simulink model "gm_PN_generator_Tx_interface"  (R2020a)
settings: Solver=FixedStepDiscrete  StartTime=0.0  StopTime=10  RelTol=1e-3  EnableMultiTasking=on
undefined symbols (not defined in the file): AXI4, Fs, ip, Lite, usb
libraries: axiinterfacelib x6, commfilt2 x4, plutoradiolib x2, commdigbbndpm3 x2, commseqgen3 x1, commutil2 x1
settings Model: Creator=juanj  LastModifiedBy=juanj
settings SolverCC: PositivePriorityOrder=on
settings OptimizationCC: BlockReduction=off  ConditionallyExecuteInputs=off  EnhancedBackFolding=on  PassReuseOutputArgsAs=Individual arguments  ZeroExternalMemoryAtStartup=off  ZeroInternalMemoryAtStartup=off  MaxStackSize=64  OptimizeBlockOrder=speed  DifferentSizesBufferReuse=on  OptimizationCustomize=off  EfficientTunableParamExpr=on
settings DebuggingCC: SignalRangeChecking=warning  AlgebraicLoopMsg=error  SingleTaskRateTransMsg=error  ParameterTunabilityLossMsg=error  UnderSpecifiedDimensionMsg=warning
settings HardwareCC: ProdBitPerPointer=32  ProdBitPerSizeT=32  ProdBitPerPtrDiffT=32  ProdLargestAtomicInteger=Long  ProdLargestAtomicFloat=Double  ProdWordSize=32  ProdLongLongMode=on  ProdHWDeviceType=ARM Compatible->ARM Cortex  TargetBitPerPointer=64  TargetBitPerSizeT=64  TargetBitPerPtrDiffT=64  TargetLongLongMode=on  TargetIntDivRoundTo=Zero  TargetEndianess=LittleEndian  TargetWordSize=64  TargetHWDeviceType=Custom Processor->MATLAB Host Computer
settings SFSimCC: MATLABDynamicMemAlloc=off
settings RTWCC: SystemTargetFile=ert.tlc  HardwareBoard=ZedBoard  TemplateMakefile=ert_default_tmf  Toolchain=Linaro AArch32 Linux v6.3.1
settings CodeAppCC: ForceParamTrailComments=on  IgnoreCustomStorageClasses=off  OperatorAnnotations=on  SimulinkDataObjDesc=on  SFDataObjDesc=on  InsertBlockDesc=on

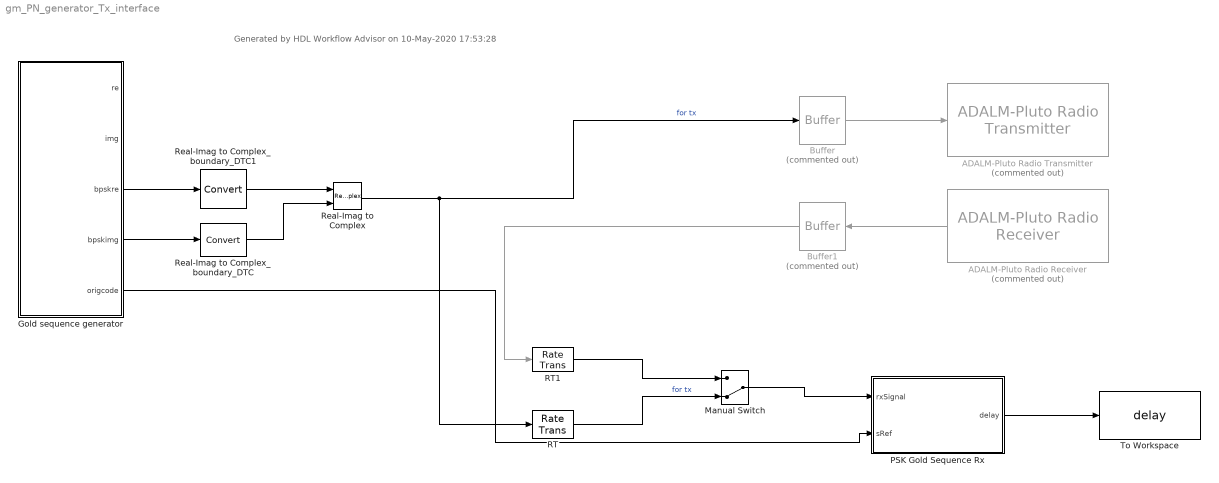
== system gm_PN_generator_Tx_interface ==
  note: Generated by HDL Workflow Advisor on 10-May-2020 17:53:28
  ADALM-Pluto Radio Receiver : plutoradiolib/ADALM-Pluto Radio Receiver  Commented=on  RadioID=usb:0  uri=ip:10.0.0.200  CenterFrequencySource=Dialog  CenterFrequency=900e6  GainSource=AGC Slow Attack  GainSourceBlock=AGC Slow Attack  Gain=10  ChannelMapping=1  BasebandSampleRate=0.5e6  OutputDataType=double  SamplesPerFrame=11216  OverflowOutputPort=off  EnableBurstMode=off  NumFramesInBurst=1  ShowAdvancedProperties=off  UseCustomFilter=off  filtPathRates=[737280000 11520000 3840000 1920000 960000 240000]  filtCoefficients=[-192 82 85 -215 228 -102 -110 290 -318 145 160 -426 471 -215 -238 633 -697 318 349 -923 1009 -457 -498 1309 -1423 640 693 -1812 1959 -876 -945 2458 -2647 1180 1268 -3290 3534 -1572 -1688 4375 -4698 2091 2247 -5836 6284 -2807 -3031 7918 -8588 3870 4225 -11182 12324 -5662 -6330 17255 -19735 9507 11312 -33568 43355 -25227 -42139 305542 305542 -42139 -25227 43355 -33568 11312 9507 -19735 17255 -6330 -5662 12324 -11182 4225 3870 -8588 7918 -3031 -2807 6284 -5836 2247 2091 -4698 4375 -1688 -1572 3534 -3290 1268 1180 -2647 2458 -945 -876 1959 -1812 693 640 -1423 1309 -498 -457 1009 -923 349 318 -697 633 -238 -215 471 -426 160 145 -318 290 -110 -102 228 -215 85 82 -192]  filtCoefficientSize=128  filtDecimInterpFactor=4  filtGain=-12  filtRFBandwidth=18000000  filterConfigStruct=struct()  EnableQuadratureCorrection=on  EnableRFDCCorrection=on  EnableBasebandDCCorrection=on  FrequencyCorrection=0  OverrideSampleTime=off  SampleTime=0.02  DataTimeout=Inf  ENSMPinControlMode=None  BISTLoopbackMode=Disabled  BISTToneInject=Disabled  BISTSignalGen=PRBS  BISTToneFreq=Fs/32  BISTToneLevel=0
      settings: SourceProductBaseCode=PLUTO
  ADALM-Pluto Radio Transmitter : plutoradiolib/ADALM-Pluto Radio Transmitter  Commented=on  RadioID=usb:0  uri=ip:10.0.0.200  CenterFrequencySource=Dialog  CenterFrequency=900e6  GainSource=Dialog  Gain=0  ChannelMapping=1  BasebandSampleRate=0.5e6  UnderflowOutputPort=off  ShowAdvancedProperties=off  UseCustomFilter=off  filtPathRates=[737280000 11520000 3840000 1920000 960000 240000]  filtCoefficients=[-192 82 85 -215 228 -102 -110 290 -318 145 160 -426 471 -215 -238 633 -697 318 349 -923 1009 -457 -498 1309 -1423 640 693 -1812 1959 -876 -945 2458 -2647 1180 1268 -3290 3534 -1572 -1688 4375 -4698 2091 2247 -5836 6284 -2807 -3031 7918 -8588 3870 4225 -11182 12324 -5662 -6330 17255 -19735 9507 11312 -33568 43355 -25227 -42139 305542 305542 -42139 -25227 43355 -33568 11312 9507 -19735 17255 -6330 -5662 12324 -11182 4225 3870 -8588 7918 -3031 -2807 6284 -5836 2247 2091 -4698 4375 -1688 -1572 3534 -3290 1268 1180 -2647 2458 -945 -876 1959 -1812 693 640 -1423 1309 -498 -457 1009 -923 349 318 -697 633 -238 -215 471 -426 160 145 -318 290 -110 -102 228 -215 85 82 -192]  filtCoefficientSize=128  filtDecimInterpFactor=4  filtGain=-12  filtRFBandwidth=18000000  filterConfigStruct=struct()  DataSourceSelect=Input Port  DDSTone1Freq=5e3  DDSTone2Freq=10e3  DDSTone1Scale=0.5  DDSTone2Scale=0.25  DataTimeout=Inf  FrequencyCorrection=0  ENSMPinControlMode=None  BISTLoopbackMode=Disabled  BISTToneInject=Disabled  BISTSignalGen=PRBS  BISTToneFreq=Fs/32  BISTToneLevel=0
      settings: SourceProductBaseCode=PLUTO
  Buffer : Buffer  Commented=on  N=11216  OutputFrames=off
  Buffer1 : Buffer  Commented=on  N=1  OutputFrames=off
  Gold sequence generator : Subsystem  TreatAsAtomicUnit=on
  Manual Switch : ManualSwitch  CurrentSetting=0
  PSK Gold Sequence Rx : Subsystem
  RT : RateTransition  OutPortSampleTime=5e-07
  RT1 : RateTransition  OutPortSampleTime=5e-07
  Real-Imag to Complex : RealImagToComplex
  Real-Imag to Complex_boundary_DTC : DataTypeConversion  SaturateOnIntegerOverflow=on  RndMeth=Zero
  Real-Imag to Complex_boundary_DTC1 : DataTypeConversion  SaturateOnIntegerOverflow=on  RndMeth=Zero
  To Workspace : ToWorkspace  VariableName=delay  SampleTime=-1
      settings: Save2DSignal=2-D array (concatenate along first dimension)
  wires:
  RT1/1 -> Manual Switch/1
  Buffer1/1 -> RT1/1
  ADALM-Pluto Radio Receiver/1 -> Buffer1/1
  RT/1 -> Manual Switch/2  "for tx"
  Manual Switch/1 -> PSK Gold Sequence Rx/1(rxSignal)
  PSK Gold Sequence Rx/1(delay) -> To Workspace/1
  Gold sequence generator/5(origcode) -> PSK Gold Sequence Rx/2(sRef)
  Real-Imag to Complex_boundary_DTC1/1 -> Real-Imag to Complex/1
  Gold sequence generator/3(bpskre) -> Real-Imag to Complex_boundary_DTC1/1
  Real-Imag to Complex_boundary_DTC/1 -> Real-Imag to Complex/2
  Gold sequence generator/4(bpskimg) -> Real-Imag to Complex_boundary_DTC/1
  Buffer/1 -> ADALM-Pluto Radio Transmitter/1
  Real-Imag to Complex/1 -> Buffer/1, RT/1  "for tx"

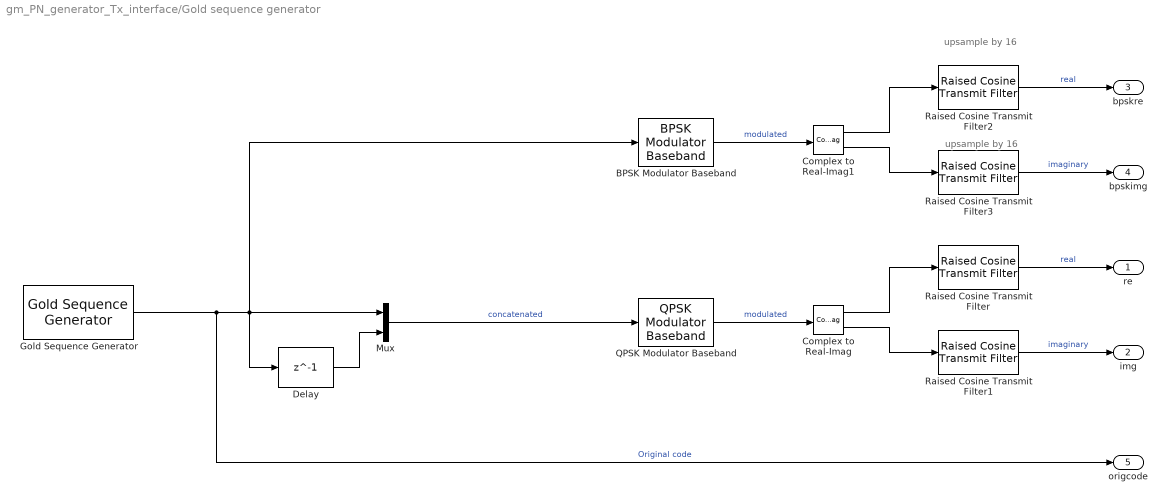
== system gm_PN_generator_Tx_interface/Gold sequence generator ==
  note: upsample by 16
  note: upsample by 16
  BPSK Modulator Baseband : commdigbbndpm3/BPSK Modulator Baseband  Ph=0  outDtype=Fixed-point  outWordLen=16  outUDDataType=sfix(16)  outFracLenMode=Best precision  outFracLen=15  outDataTypeStr=fixdt(1,16)  outLastDataTypeStr=fixdt(1,16)
  Complex to Real-Imag : ComplexToRealImag
  Complex to Real-Imag1 : ComplexToRealImag
  Delay : Delay  DelayLength=1  InitialCondition=0  UseCircularBuffer=on
  Gold Sequence Generator : commseqgen3/Gold Sequence Generator  genPoly1='z^6 + z + 1'  iniState1=[0 1 0 1 0 1]  genPoly2='z^6 + z^5 + z^2 + z + 1'  iniState2=[0 0 0 0 0 1]  index=0  shift=0  outVarSiz=off  maxOutSizeMode=Dialog parameter  maxOutSize=[10 1]  Ts=1/5000  sampPerFrame=1  reset=off  outDataType=boolean
      settings: SourceProductBaseCode=CM
  Mux : Mux  Inputs=2
  QPSK Modulator Baseband : commdigbbndpm3/QPSK Modulator Baseband  InType=Bit  Enc=Gray  Ph=pi/4  outDtype=Fixed-point  outWordLen=16  outUDDataType=sfix(16)  outFracLenMode=Best precision  outFracLen=15  outDataTypeStr=fixdt(1,16)  outLastDataTypeStr=fixdt(1,16)
  Raised Cosine Transmit Filter : commfilt2/Raised Cosine Transmit Filter  filtType=Square root  R=0.7  filtSpan=12  N=2  filterGain=1  RateOptions=Allow multirate processing  framing=Mute  checkCoeff=off  variableName=rcTxFilt  checkGain=Normalized  sampMode=Mute  saveAsFlag=0  currentFiltSpan=12  D=(12)/2  launchFVT=on  roundingMode=Floor  overflowMode=off  coeffDataTypeStr=Inherit: Same word length as input  coeffMin=[]  coeffMax=[]  coeffLastDataTypeStr=Inherit: Same word length as input  outputMin=[]  outputMax=[]
  Raised Cosine Transmit Filter1 : commfilt2/Raised Cosine Transmit Filter  filtType=Square root  R=0.7  filtSpan=12  N=2  filterGain=1  RateOptions=Allow multirate processing  framing=Mute  checkCoeff=off  variableName=rcTxFilt1  checkGain=Normalized  sampMode=Mute  saveAsFlag=0  currentFiltSpan=12  D=(12)/2  launchFVT=on  roundingMode=Floor  overflowMode=off  coeffDataTypeStr=Inherit: Same word length as input  coeffMin=[]  coeffMax=[]  coeffLastDataTypeStr=Inherit: Same word length as input  outputMin=[]  outputMax=[]
  Raised Cosine Transmit Filter2 : commfilt2/Raised Cosine Transmit Filter  filtType=Square root  R=0.5  filtSpan=10  N=16  filterGain=1  InputProcessing=Columns as channels (frame based)  RateOptions=Allow multirate processing  framing=Mute  checkCoeff=off  variableName=rcTxFilt2  checkGain=Normalized  sampMode=Mute  saveAsFlag=0  currentFiltSpan=10  D=(10)/2  launchFVT=on  roundingMode=Floor  overflowMode=off  coeffDataTypeStr=Inherit: Same word length as input  coeffMin=[]  coeffMax=[]  coeffLastDataTypeStr=Inherit: Same word length as input  outputMin=[]  outputMax=[]
  Raised Cosine Transmit Filter3 : commfilt2/Raised Cosine Transmit Filter  filtType=Square root  R=0.5  filtSpan=10  N=16  filterGain=1  InputProcessing=Columns as channels (frame based)  RateOptions=Allow multirate processing  framing=Mute  checkCoeff=off  variableName=rcTxFilt3  checkGain=Normalized  sampMode=Mute  saveAsFlag=0  currentFiltSpan=10  D=(10)/2  launchFVT=on  roundingMode=Floor  overflowMode=off  coeffDataTypeStr=Inherit: Same word length as input  coeffMin=[]  coeffMax=[]  coeffLastDataTypeStr=Inherit: Same word length as input  outputMin=[]  outputMax=[]
  re : Outport
  img : Outport  Port=2  VectorParamsAs1DForOutWhenUnconnected=off
  bpskre : Outport  Port=3
  bpskimg : Outport  Port=4  VectorParamsAs1DForOutWhenUnconnected=off
  origcode : Outport  Port=5
  wires:
  BPSK Modulator Baseband/1 -> Complex to Real-Imag1/1  "modulated"
  Complex to Real-Imag1/2 -> Raised Cosine Transmit Filter3/1
  Raised Cosine Transmit Filter2/1 -> bpskre/1  "real"
  Raised Cosine Transmit Filter3/1 -> bpskimg/1  "imaginary"
  Complex to Real-Imag1/1 -> Raised Cosine Transmit Filter2/1
  Delay/1 -> Mux/2
  Mux/1 -> QPSK Modulator Baseband/1  "concatenated"
  Gold Sequence Generator/1 -> Mux/1, BPSK Modulator Baseband/1, Delay/1, origcode/1  "Original code"
  Complex to Real-Imag/2 -> Raised Cosine Transmit Filter1/1
  Complex to Real-Imag/1 -> Raised Cosine Transmit Filter/1
  Raised Cosine Transmit Filter1/1 -> img/1  "imaginary"
  Raised Cosine Transmit Filter/1 -> re/1  "real"
  QPSK Modulator Baseband/1 -> Complex to Real-Imag/1  "modulated"

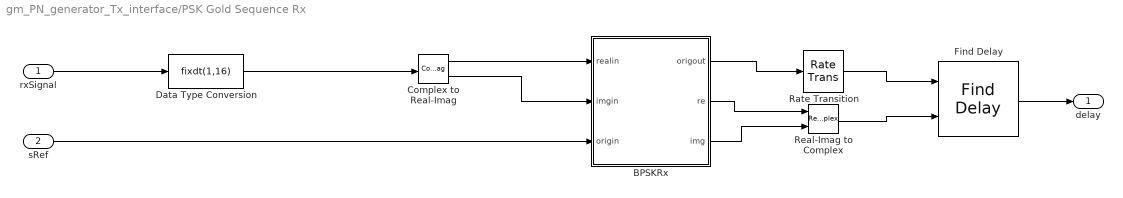
== system gm_PN_generator_Tx_interface/PSK Gold Sequence Rx ==
  rxSignal : Inport
  sRef : Inport  Port=2
  BPSKRx : Subsystem  TreatAsAtomicUnit=on  mask(AXI4-Lite/AXI4 Interface){}
      mask help:
      | This is an automatically generated subsystem block.
      | This contains the AXI interface blocks that communicate with the GoldSeque_ip IPCore generated from PN_generator_Tx/PSK Gold Sequence Rx/BPSKRx subsystem.
      mask Display: disp(sprintf('Xilinx Zynq \nAXI Interface'));
  Complex to Real-Imag : ComplexToRealImag
  Data Type Conversion : DataTypeConversion  OutMax=[1]  OutDataTypeStr=fixdt(1,16)
  Find Delay : commutil2/Find Delay  corrLength=200  chgSigOP=off  stopUpdate=off  numConstDelay=3
      settings: SourceProductBaseCode=CM
  Rate Transition : RateTransition
  Real-Imag to Complex : RealImagToComplex
  delay : Outport
  wires:
  Complex to Real-Imag/1 -> BPSKRx/1(realin)
  Complex to Real-Imag/2 -> BPSKRx/2(imgin)
  Data Type Conversion/1 -> Complex to Real-Imag/1
  Real-Imag to Complex/1 -> Find Delay/2
  BPSKRx/3(img) -> Real-Imag to Complex/2
  BPSKRx/2(re) -> Real-Imag to Complex/1
  Rate Transition/1 -> Find Delay/1
  BPSKRx/1(origout) -> Rate Transition/1
  sRef/1 -> BPSKRx/3(origin)
  rxSignal/1 -> Data Type Conversion/1
  Find Delay/1 -> delay/1

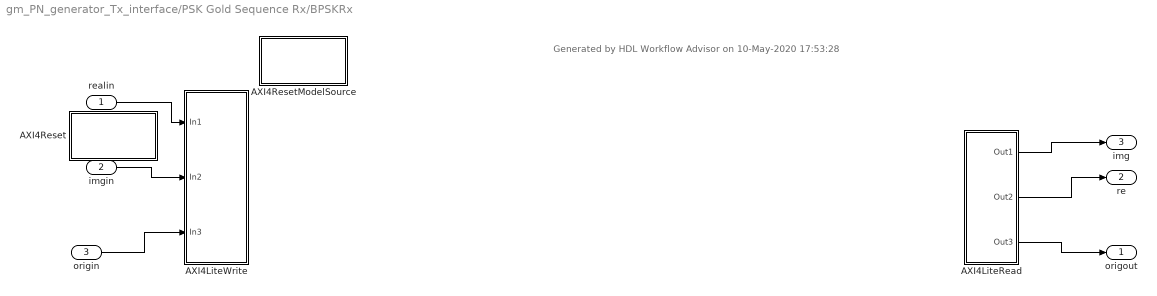
== system gm_PN_generator_Tx_interface/PSK Gold Sequence Rx/BPSKRx ==
  note: Generated by HDL Workflow Advisor on 10-May-2020 17:53:28
  realin : Inport
  imgin : Inport  Port=2
  origin : Inport  Port=3
  AXI4LiteRead : Subsystem  Priority=10
  AXI4LiteWrite : Subsystem  Priority=1
  AXI4Reset : Subsystem  mask(System Start){ShowInLibBrowser=0}
      mask prompts: ShowInLibBrowser "Simulink:masks:CustCodeMaskParam1_MP"
      settings: CopyFcn=cccopyfcn(gcb)  OpenFcn=ccopenfcn('System Start Function')
      mask Help: eval('feval(''rtwprivate'',''rtwhelpview'',''rtw_sys_start_block'')');
      mask Display: disp('System\nStart');
  AXI4ResetModelSource : Subsystem  mask(Model Source){ShowInLibBrowser=0}
      mask prompts: ShowInLibBrowser "Simulink:masks:CustCodeMaskParam1_MP"
      settings: CopyFcn=cccopyfcn(gcb)  OpenFcn=ccopenfcn('Model Source')
      mask Help: eval('feval(''rtwprivate'',''rtwhelpview'',''rtw_model_source_block'')');
      mask Display: disp('Model\nSource');
  origout : Outport
  re : Outport  Port=2
  img : Outport  Port=3
  wires:
  realin/1 -> AXI4LiteWrite/1(In1)
  imgin/1 -> AXI4LiteWrite/2(In2)
  origin/1 -> AXI4LiteWrite/3(In3)
  AXI4LiteRead/1(Out1) -> img/1
  AXI4LiteRead/2(Out2) -> re/1
  AXI4LiteRead/3(Out3) -> origout/1

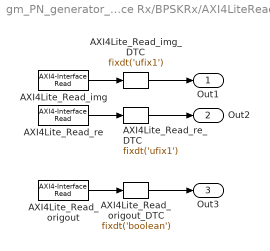
== system gm_PN_generator_Tx_interface/PSK Gold Sequence Rx/BPSKRx/AXI4LiteRead ==
  AXI4Lite_Read_img : axiinterfacelib/AXI4-Interface Read  Priority=4  AXIInterfaceType=AXI4-Lite  DeviceName=/dev/mwipcore  RegisterOffset=hex2dec('114')  DataLength=1  DataType=uint32  SampleTime=-1  blockPlatform=ZYNQ  SimulateUsing=Interpreted Execution
      settings: SourceProductBaseCode=ECZYNQ7000
  AXI4Lite_Read_img_DTC : DataTypeConversion  OutDataTypeStr=fixdt('ufix1')  ConvertRealWorld=Stored Integer (SI)
  AXI4Lite_Read_origout : axiinterfacelib/AXI4-Interface Read  Priority=2  AXIInterfaceType=AXI4-Lite  DeviceName=/dev/mwipcore  RegisterOffset=hex2dec('10C')  DataLength=1  DataType=uint32  SampleTime=-1  blockPlatform=ZYNQ  SimulateUsing=Interpreted Execution
      settings: SourceProductBaseCode=ECZYNQ7000
  AXI4Lite_Read_origout_DTC : DataTypeConversion  OutDataTypeStr=fixdt('boolean')  ConvertRealWorld=Stored Integer (SI)
  AXI4Lite_Read_re : axiinterfacelib/AXI4-Interface Read  Priority=3  AXIInterfaceType=AXI4-Lite  DeviceName=/dev/mwipcore  RegisterOffset=hex2dec('110')  DataLength=1  DataType=uint32  SampleTime=-1  blockPlatform=ZYNQ  SimulateUsing=Interpreted Execution
      settings: SourceProductBaseCode=ECZYNQ7000
  AXI4Lite_Read_re_DTC : DataTypeConversion  OutDataTypeStr=fixdt('ufix1')  ConvertRealWorld=Stored Integer (SI)
  Out1 : Outport
  Out2 : Outport  Port=2
  Out3 : Outport  Port=3
  wires:
  AXI4Lite_Read_re_DTC/1 -> Out2/1
  AXI4Lite_Read_origout/1 -> AXI4Lite_Read_origout_DTC/1
  AXI4Lite_Read_img/1 -> AXI4Lite_Read_img_DTC/1
  AXI4Lite_Read_img_DTC/1 -> Out1/1
  AXI4Lite_Read_re/1 -> AXI4Lite_Read_re_DTC/1
  AXI4Lite_Read_origout_DTC/1 -> Out3/1

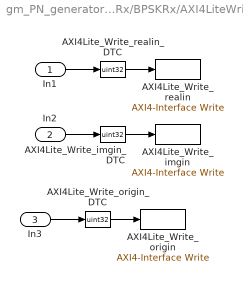
== system gm_PN_generator_Tx_interface/PSK Gold Sequence Rx/BPSKRx/AXI4LiteWrite ==
  In1 : Inport
  In2 : Inport  Port=2
  In3 : Inport  Port=3
  AXI4Lite_Write_imgin : axiinterfacelib/AXI4-Interface Write  Priority=2  AXIInterfaceType=AXI4-Lite  DeviceName=/dev/mwipcore  RegisterOffset=hex2dec('104')  blockPlatform=ZYNQ  SimulateUsing=Interpreted execution
      settings: SourceProductBaseCode=ECZYNQ7000
  AXI4Lite_Write_imgin_DTC : DataTypeConversion  OutDataTypeStr=uint32  ConvertRealWorld=Stored Integer (SI)
  AXI4Lite_Write_origin : axiinterfacelib/AXI4-Interface Write  Priority=3  AXIInterfaceType=AXI4-Lite  DeviceName=/dev/mwipcore  RegisterOffset=hex2dec('108')  blockPlatform=ZYNQ  SimulateUsing=Interpreted execution
      settings: SourceProductBaseCode=ECZYNQ7000
  AXI4Lite_Write_origin_DTC : DataTypeConversion  OutDataTypeStr=uint32  ConvertRealWorld=Stored Integer (SI)
  AXI4Lite_Write_realin : axiinterfacelib/AXI4-Interface Write  Priority=1  AXIInterfaceType=AXI4-Lite  DeviceName=/dev/mwipcore  RegisterOffset=hex2dec('100')  blockPlatform=ZYNQ  SimulateUsing=Interpreted execution
      settings: SourceProductBaseCode=ECZYNQ7000
  AXI4Lite_Write_realin_DTC : DataTypeConversion  OutDataTypeStr=uint32  ConvertRealWorld=Stored Integer (SI)
  wires:
  AXI4Lite_Write_origin_DTC/1 -> AXI4Lite_Write_origin/1
  AXI4Lite_Write_realin_DTC/1 -> AXI4Lite_Write_realin/1
  In1/1 -> AXI4Lite_Write_realin_DTC/1
  AXI4Lite_Write_imgin_DTC/1 -> AXI4Lite_Write_imgin/1
  In3/1 -> AXI4Lite_Write_origin_DTC/1
  In2/1 -> AXI4Lite_Write_imgin_DTC/1

== system gm_PN_generator_Tx_interface/PSK Gold Sequence Rx/BPSKRx/AXI4Reset ==

== system gm_PN_generator_Tx_interface/PSK Gold Sequence Rx/BPSKRx/AXI4ResetModelSource ==
